simulink model "BatteryHV_harness_model"  (R2022a)
settings: Solver=daessc  StartTime=0.0  StopTime=t_end  RelTol=1e-3
PreLoadFcn:
  | BatteryHV_harness_setup
undefined symbols (not defined in the file or in its folder): Minus, Plus
libraries: fl_lib x6, nesl_utility x5
settings Model: Creator=isaacito  LastModifiedBy=isaacito
settings DataIOCC: DSMLogging=off
settings SimscapeCC: SimscapeLogType=all  SimscapeLogSimulationStatistics=on  SimscapeLogLimitData=off

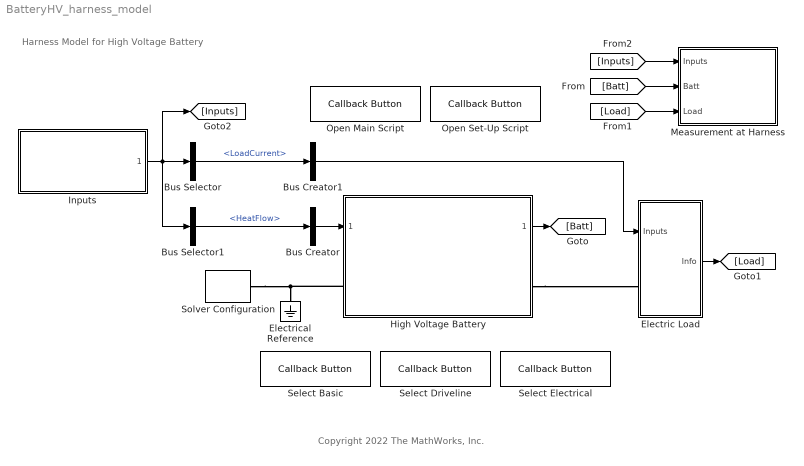
== system BatteryHV_harness_model ==
  note: Harness Model for High Voltage Battery
  note: Copyright 2022 The MathWorks, Inc.
  Bus Creator : BusCreator  Inputs=1
  Bus Creator1 : BusCreator  Inputs=1
  Bus Selector : BusSelector  OutputSignals=LoadCurrent
  Bus Selector1 : BusSelector  OutputSignals=HeatFlow
  Electric Load : Subsystem
  Electrical Reference : fl_lib/Electrical/Electrical Elements/Electrical Reference
      settings: SourceProductBaseCode=PW,SS,VE
  High Voltage Battery : Subsystem  ReferencedSubsystem=BatteryHV_refsub_Driveline
  Inputs : Subsystem  ReferencedSubsystem=BatteryHV_input_refsub
  Measurement at Harness : Subsystem
  Open Main Script : CallbackButton  ButtonText=Open Main Script
      settings: ClickFcn=edit BatteryhV_main_script
  Open Set-Up Script : CallbackButton  ButtonText=Open Set-Up Script
      settings: ClickFcn=edit BatteryHV_harness_setup
  Select Basic : CallbackButton  ButtonText=Select
      settings: ClickFcn=|
      | blk = gcs + "/High Voltage Battery";
      | set_param( blk, ...
      |     ReferencedSubsystem = ...
      |     "BatteryHV_refsub_Basic" );
      | 
      | % Fit the system to the window.
      | % This centers the system.
      | set_param(blk, ZoomFactor='FitSystem')
      | % Then set the zoom factor to 100%.
      | set_param(blk, ZoomFactor='100')
  Select Driveline : CallbackButton  ButtonText=Select
      settings: ClickFcn=|
      | blk = gcs + "/High Voltage Battery";
      | set_param( blk, ...
      |     ReferencedSubsystem = ...
      |     "BatteryHV_refsub_Driveline" );
      | 
      | % Fit the system to the window.
      | % This centers the system.
      | set_param(blk, ZoomFactor='FitSystem')
      | % Then set the zoom factor to 100%.
      | set_param(blk, ZoomFactor='100')
  Select Electrical : CallbackButton  ButtonText=Select
      settings: ClickFcn=|
      | blk =  gcs + "/High Voltage Battery";
      | set_param( blk, ...
      |     ReferencedSubsystem = ...
      |     "BatteryHV_refsub_Electrical" );
      | 
      | % Fit the system to the window.
      | % This centers the system.
      | set_param(blk, ZoomFactor='FitSystem')
      | % Then set the zoom factor to 100%.
      | set_param(blk, ZoomFactor='100')
  Solver Configuration : nesl_utility/Solver Configuration  PhysicalDomain=network_engine_domain  SubClassName=solver  LeftPortType=input  RightPortType=generic  Tones=[]  Harmonics=[]  SimulateNoise=off  Profile=off  UseLocalSampling=off  EnableSwitchedLinearOptims=on  FrequencyDomain=off  UseCCode=off  RelTol=0.001  AbsTol=0.001  MinStep=1e-09  ToWorkspace=off  RevertToSquareIcSolve=off  NumHomotopyIterations=100  PhasorMode=off  PhasorModeNumHarmonics=1  IndexReductionMethod=DerivativeReplacement  DoDC=off  ResidualTolerance=1e-09  UseLocalSolver=off  LocalSolverChoice=NE_BACKWARD_EULER_ADVANCER  LocalSolverSampleTime=0.001  DoFixedCost=off  MaxNonlinIter=3  MaxModeIter=2  ComputeImpulses=off  ImpulseIterations=2  LinearAlgebra=auto  LinearAlgebraNumThread=0  EquationFormulation=NE_TIME_EF  DelaysMemoryBudget=1024  AutomaticFiltering=on  FilteringTimeConstant=0.001  PartitionStorageMethod=AS_NEEDED  PartitionMemoryBudget=1024  PartitionMethod=ROBUST
      settings: AttributesFormatString=Local solver: %<UseLocalSolver>  SourceProductBaseCode=SS,PW,VE
  wires:
  Bus Creator/1 -> High Voltage Battery/1
  High Voltage Battery/1 -> [Batt]
  [Batt] -> Measurement at Harness/2(Batt)
  Electric Load/1(Info) -> [Load]
  [Load] -> Measurement at Harness/3(Load)
  Bus Creator1/1 -> Electric Load/1(Inputs)
  Inputs/1 -> Bus Selector1/1, [Inputs], Bus Selector/1
  Bus Selector/1 -> Bus Creator1/1  "<LoadCurrent>"
  [Inputs] -> Measurement at Harness/1(Inputs)
  Bus Selector1/1 -> Bus Creator/1  "<HeatFlow>"
  connections:
  High Voltage Battery/LConn1 -- Electrical Reference/LConn1 -- Solver Configuration/RConn1
  High Voltage Battery/RConn1 -- Electric Load/LConn1

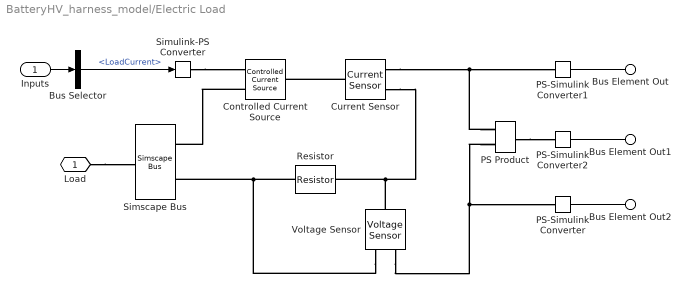
== system BatteryHV_harness_model/Electric Load ==
  Inputs : Inport
  Bus Selector : BusSelector  OutputSignals=LoadCurrent
  Controlled Current Source : fl_lib/Electrical/Electrical Sources/Controlled Current Source
      settings: SourceProductBaseCode=PW,SS,VE
  Current Sensor : fl_lib/Electrical/Electrical Sensors/Current Sensor
      settings: SourceProductBaseCode=PW,SS,VE
  PS Product : fl_lib/Physical Signals/Functions/PS Product
      settings: SourceProductBaseCode=PW,SS,VE
  PS-Simulink Converter : nesl_utility/PS-Simulink Converter  PhysicalDomain=network_engine_domain  SubClassName=ps_output  LeftPortType=input  RightPortType=output  PseudoPeriodic=off  Frequencies=[]  VectorFormat=inherit  Unit=V  AffineConversion=off
      settings: SourceProductBaseCode=SS,PW,VE
  PS-Simulink Converter1 : nesl_utility/PS-Simulink Converter  PhysicalDomain=network_engine_domain  SubClassName=ps_output  LeftPortType=input  RightPortType=output  PseudoPeriodic=off  Frequencies=[]  VectorFormat=inherit  Unit=A  AffineConversion=off
      settings: SourceProductBaseCode=SS,PW,VE
  PS-Simulink Converter2 : nesl_utility/PS-Simulink Converter  PhysicalDomain=network_engine_domain  SubClassName=ps_output  LeftPortType=input  RightPortType=output  PseudoPeriodic=off  Frequencies=[]  VectorFormat=inherit  Unit=kW  AffineConversion=off
      settings: SourceProductBaseCode=SS,PW,VE
  Resistor : fl_lib/Electrical/Electrical Elements/Resistor  R=1 Ohm  i_specify=off  i_priority=None  i=0 A  i_nominal_specify=off  i_nominal_unit=A  i_nominal_value=1  v_specify=off  v_priority=None  v=0 V  v_nominal_specify=off  v_nominal_unit=V  v_nominal_value=1
      settings: SourceProductBaseCode=PW,SS,VE
  Simscape Bus : SimscapeBus  HierarchyStrings=Plus;Minus  ConnectionType=Bus: Bus_HighVoltage
      settings: AttributesFormatString=%<ConnectionType>
  Simulink-PS Converter : nesl_utility/Simulink-PS Converter  PhysicalDomain=network_engine_domain  SubClassName=ps_input  LeftPortType=input  RightPortType=output  PseudoPeriodic=off  Frequencies=[]  NoiseDistribution=none  NoiseParameters=[]  Unit=A  AffineConversion=off  FilteringAndDerivatives=provide  SimscapeFilterOrder=1  InputFilterTimeConstant=0.001  UdotUserProvided=0
      settings: SourceProductBaseCode=SS,PW,VE
  Voltage Sensor : fl_lib/Electrical/Electrical Sensors/Voltage Sensor
      settings: SourceProductBaseCode=PW,SS,VE
  Load : PMIOPort  Side=Left
  Bus Element Out : Outport  PortName=Info  Element=Curr
  Bus Element Out1 : Outport  PortName=Info  Element=Pwr
  Bus Element Out2 : Outport  PortName=Info  Element=V
  wires:
  PS-Simulink Converter1/1 -> Bus Element Out/1
  PS-Simulink Converter2/1 -> Bus Element Out1/1
  PS-Simulink Converter/1 -> Bus Element Out2/1
  Inputs/1 -> Bus Selector/1
  Bus Selector/1 -> Simulink-PS Converter/1  "<LoadCurrent>"
  connections:
  Load/RConn1 -- Simscape Bus/RConn1
  Controlled Current Source/RConn2 -- Simscape Bus/LConn1
  Resistor/RConn1 -- Voltage Sensor/RConn2 -- Simscape Bus/LConn2
  Simulink-PS Converter/RConn1 -- Controlled Current Source/RConn1
  Current Sensor/LConn1 -- Controlled Current Source/LConn1
  Current Sensor/RConn2 -- Resistor/LConn1 -- Voltage Sensor/LConn1
  Voltage Sensor/RConn1 -- PS Product/LConn2 -- PS-Simulink Converter/LConn1
  Current Sensor/RConn1 -- PS-Simulink Converter1/LConn1 -- PS Product/LConn1
  PS Product/RConn1 -- PS-Simulink Converter2/LConn1

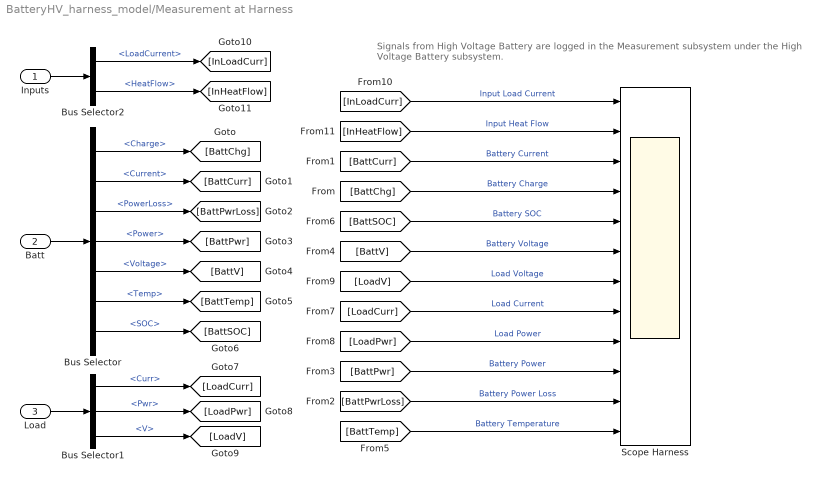
== system BatteryHV_harness_model/Measurement at Harness ==
  note: Signals from High Voltage Battery are logged in
      | the Measurement subsystem under the High Voltage Battery subsystem.
  Inputs : Inport
  Batt : Inport  Port=2
  Load : Inport  Port=3
  Bus Selector : BusSelector  OutputSignals=Charge,Current,PowerLoss,Power,Voltage,Temp,SOC
  Bus Selector1 : BusSelector  OutputSignals=Curr,Pwr,V
  Bus Selector2 : BusSelector  OutputSignals=LoadCurrent,HeatFlow
  Scope Harness : Scope  NumInputPorts=12
  wires:
  Batt/1 -> Bus Selector/1
  Bus Selector/1 -> [BattChg]  "<Charge>"
  Bus Selector/2 -> [BattCurr]  "<Current>"
  Bus Selector/3 -> [BattPwrLoss]  "<PowerLoss>"
  Bus Selector/4 -> [BattPwr]  "<Power>"
  Bus Selector/5 -> [BattV]  "<Voltage>"
  Bus Selector/6 -> [BattTemp]  "<Temp>"
  Bus Selector/7 -> [BattSOC]  "<SOC>"
  Load/1 -> Bus Selector1/1
  Bus Selector1/1 -> [LoadCurr]  "<Curr>"
  Bus Selector1/2 -> [LoadPwr]  "<Pwr>"
  Bus Selector1/3 -> [LoadV]  "<V>"
  [BattCurr] -> Scope Harness/3  "Battery Current"
  [BattChg] -> Scope Harness/4  "Battery Charge"
  [BattSOC] -> Scope Harness/5  "Battery SOC"
  [BattV] -> Scope Harness/6  "Battery Voltage"
  [LoadV] -> Scope Harness/7  "Load Voltage"
  [LoadCurr] -> Scope Harness/8  "Load Current"
  [LoadPwr] -> Scope Harness/9  "Load Power"
  [BattPwr] -> Scope Harness/10  "Battery Power"
  [BattPwrLoss] -> Scope Harness/11  "Battery Power Loss"
  [BattTemp] -> Scope Harness/12  "Battery Temperature"
  Inputs/1 -> Bus Selector2/1
  Bus Selector2/1 -> [InLoadCurr]  "<LoadCurrent>"
  [InLoadCurr] -> Scope Harness/1  "Input Load Current"
  Bus Selector2/2 -> [InHeatFlow]  "<HeatFlow>"
  [InHeatFlow] -> Scope Harness/2  "Input Heat Flow"
